simulink model "model"  (R2024b)
settings: Solver=ode4  StartTime=0.0  StopTime=tfinal  FixedStep=dt  RelTol=1e-3
values from neighbouring files (symbols this model uses):
  A_lateral = [YV , (W0+YP) , -U0+YR, g*cos(theta0), 0;         LV_DASH , LP_DASH , LR_DASH , 0 , 0;         NV_DASH , NP_DASH , NR_DASH , 0 , 0;         0 , 1 , tan(theta0) , 0 , 0;         0 , 0 , 1/cos(theta0) ,0 ,0]    [pre_simulink.m]
  A_longitudinal = [XU,XW,-W0,-g*cos(theta0);         ZU/(1-ZWD),ZW/(1-ZWD),(ZQ+U0)/(1-ZWD),-g*sin(theta0)/(1-ZWD);         MU+MWD*ZU/(1-ZWD),MW+MWD*ZW/(1-ZWD),MQ+MWD*(ZQ+U0)/(1-ZWD),-MWD*g*sin(theta0)/(1-ZWD);         0,0,1,0]    [pre_simulink.m]
  B_lateral = [YDA , YDR;          LDA_DASH , LDR_DASH;          NDA_DASH , NDR_DASH;          0 , 0;          0 , 0]    [pre_simulink.m]
  B_longitudinal = [XDE,XDTH ;         ZDE/(1-ZWD),ZDTH/(1-ZWD);         MDE+MWD*ZDE/(1-ZWD),MDTH+MWD*ZDTH/(1-ZWD);         0,0]    [pre_simulink.m]
  C_lateral = eye(5)    [pre_simulink.m]
  C_longitudinal = eye(4)    [pre_simulink.m]
  Controls_Matrix = [0,    XDE,   XDTH,      0 ... (first row only)    [aircraft_data_reader.m]
  D_lateral = zeros(5,2)    [pre_simulink.m]
  D_longitudinal = zeros(4,2)    [pre_simulink.m]
  dA = 0 *pi/180    (= 0)    [pre_simulink.m]
  dR = 0 *pi/180    (= 0)    [pre_simulink.m]
  dTH = 0    [pre_simulink.m]
  g = aircraft_data(52)    [aircraft_data_reader.m]
  Ixx = aircraft_data(53)    [aircraft_data_reader.m]
  Iyy = aircraft_data(54)    [aircraft_data_reader.m]
  Izz = aircraft_data(55)    [aircraft_data_reader.m]
  K = 1.5849    [pre_simulink.m]
  K_d_theta = 0.9182    [pre_simulink.m]
  K_i = 0.0332    [pre_simulink.m]
  m = aircraft_data(51)    [aircraft_data_reader.m]
  mg0 = m*g * [ sin(s0(8)) ; -cos(s0(8))*sin(s0(7)) ; -cos(s0(8))*cos(s0(7)) ]    [aircraft_data_reader.m]
  s0 = aircraft_data(4:15)    [aircraft_data_reader.m]
  States_Matrix = [XU,   0,   XW,    0,   0,   0,    0 ... (first row only)    [aircraft_data_reader.m]
  U0 = s0(1)    [aircraft_data_reader.m]
undefined symbols (not defined in the file or in its folder): A_lateral_1DOF, A_lateral_2DOF, A_lateral_3DOF_DR, A_lateral_3DOF_SP, A_longitudinal_lp, A_longitudinal_sp, alpha, B_lateral_1DOF, B_lateral_2DOF, B_lateral_3DOF_DR, B_lateral_3DOF_SP, B_longitudinal_lp, B_longitudinal_sp, beta, C_lateral_1DOF, C_lateral_2DOF, C_lateral_3DOF_DR, C_lateral_3DOF_SP, C_longitudinal_lp, C_longitudinal_sp, d_a, d_e, D_lateral_1DOF, D_lateral_2DOF, D_lateral_3DOF_DR, D_lateral_3DOF_SP, D_longitudinal_lp, D_longitudinal_sp, d_r, d_th, initial_states_bus, p, phi, psi, q, r, theta, v, VT, w, wdot, x, y, z
libraries: cstblocks x4, dspsigops x3, simulink_extras x1, shared6dof x1, aerolibasang x1
settings Model: Creator=ahmed  LastModifiedBy=ahmed
settings DebuggingCC: SignalInfNanChecking=warning  CheckMatrixSingularityMsg=warning  SignalLabelMismatchMsg=warning  StateNameClashWarn=warning

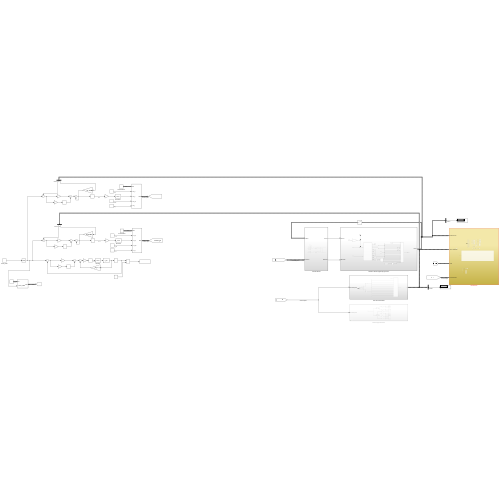
[thumbnail: Simulink's stored preview of the top-level diagram]
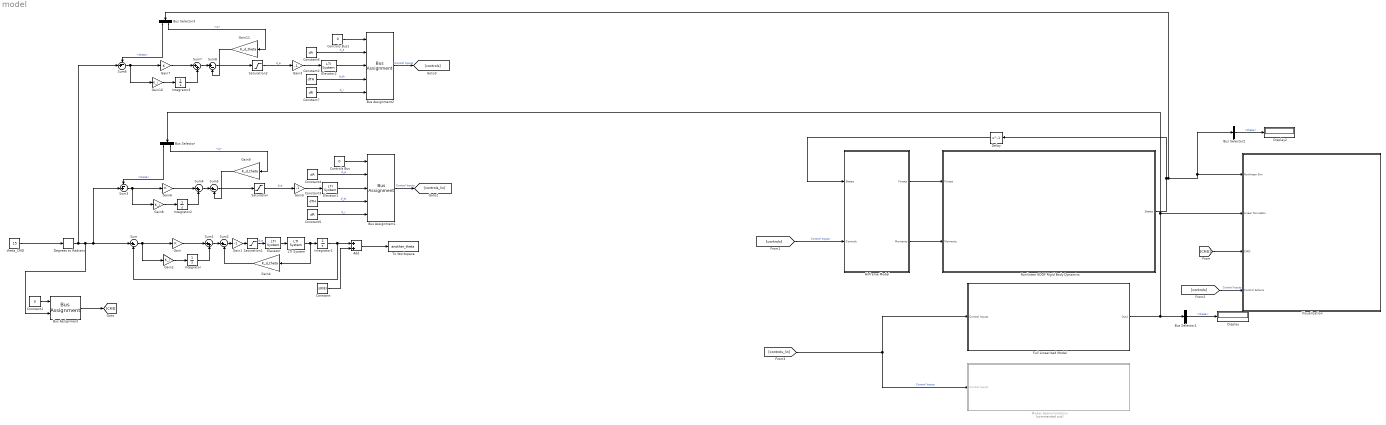
== system model ==
  Add : Sum
  Airframe Model : Subsystem
  Bus Assignment : BusAssignment  AssignedSignals=theta_CMD
  Bus Assignment1 : BusAssignment  AssignedSignals=d_a,d_e,d_th,d_r
  Bus Assignment2 : BusAssignment  AssignedSignals=d_a,d_e,d_th,d_r
  Bus Selector : BusSelector  OutputSignals=theta,q
  Bus Selector1 : BusSelector  OutputSignals=theta
  Bus Selector2 : BusSelector  OutputSignals=theta
  Bus Selector3 : BusSelector  OutputSignals=theta,q
  Constant : Constant  Value=s0(8)
  Constant1 : Constant  Value=0  OutDataTypeStr=Bus: CMD_States_bus_T
  Constant2 : Constant  Value=dTH
  Constant3 : Constant  Value=dTH
  Constant4 : Constant  Value=dA
  Constant5 : Constant  Value=dR
  Constant6 : Constant  Value=dA
  Constant7 : Constant  Value=dR
  Controls Bus : Constant  Value=0  OutDataTypeStr=Bus: Controls_bus_T
  Controls Bus1 : Constant  Value=0  OutDataTypeStr=Bus: Controls_bus_T
  Degrees to Radians : simulink_extras/Transformations/Degrees to Radians
  Delay : Delay  DelayLength=1  InitialCondition=initial_states_bus
  Display : Display
  Display2 : Display
  Elevator : cstblocks/LTI System  sys=servo  IC=[]  PadeOrder=0
  Elevator1 : cstblocks/LTI System  sys=servo  IC=[]  PadeOrder=0
  Elevator2 : cstblocks/LTI System  sys=servo  IC=[]  PadeOrder=0
  Full Linearized Model : Subsystem
  Gain : Gain  Gain=K
  Gain1 : Gain  Gain=-1
  Gain10 : Gain  Gain=K_i
  Gain11 : Gain  Gain=K_d_theta
  Gain2 : Gain  Gain=K_i
  Gain3 : Gain  Gain=-1
  Gain4 : Gain  Gain=K_d_theta
  Gain5 : Gain  Gain=-1
  Gain6 : Gain  Gain=K
  Gain7 : Gain  Gain=K
  Gain8 : Gain  Gain=K_i
  Gain9 : Gain  Gain=K_d_theta
  Integrator{,1..3} (4 alike) : Integrator
  LTI System : cstblocks/LTI System  sys=q_de  IC=[]  PadeOrder=0
  Modes Approximations : Subsystem  Commented=on
  Nonlinear 6DOF Rigid Body Dynamics : Subsystem
  Saturation : Saturate  UpperLimit=30*pi/180  LowerLimit=-30*pi/180
  Saturation1 : Saturate  UpperLimit=30*pi/180  LowerLimit=-30*pi/180
  Saturation2 : Saturate  UpperLimit=30*pi/180  LowerLimit=-30*pi/180
  Sum{,2,5,8} (4 alike) : Sum  Inputs=|+-
  Sum1 : Sum  Inputs=|++
  Sum3 : Sum  Inputs=-+|
  Sum4 : Sum  Inputs=|++
  Sum6 : Sum  Inputs=-+|
  Sum7 : Sum  Inputs=|++
  To Workspace : ToWorkspace  VariableName=another_theta  SaveFormat=Timeseries  SampleTime=-1
  Visualization : Subsystem
  theta_CMD : Constant  Value=15
  wires:
  Airframe Model/1(Forces) -> Nonlinear 6DOF Rigid Body Dynamics/1(Forces)
  Airframe Model/2(Moments) -> Nonlinear 6DOF Rigid Body Dynamics/2(Moments)
  Delay/1 -> Airframe Model/1(States)
  Bus Selector/1 -> Sum3/1  "<theta>"
  Gain1/1 -> Saturation1/1
  Integrator/1 -> Sum1/2
  Sum1/1 -> Sum2/1
  Gain2/1 -> Integrator/1
  Full Linearized Model/1(Out1) -> Visualization/2(Linear Simulator), Bus Selector/1, Bus Selector1/1
  Gain/1 -> Sum1/1
  LTI System/1 -> Gain4/1, Integrator1/1
  Integrator1/1 -> Sum/2, Add/1
  theta_CMD/1 -> Degrees to Radians/1
  Gain4/1 -> Sum2/2
  [controls] -> Airframe Model/2(Controls)  "Control Inputs"
  Constant4/1 -> Bus Assignment1/2  "d_a"
  Constant3/1 -> Bus Assignment1/4  "d_th"
  Elevator/1 -> LTI System/1
  Constant5/1 -> Bus Assignment1/5  "d_r"
  Controls Bus/1 -> Bus Assignment1/1
  Saturation/1 -> Gain5/1  "d_e"
  Gain5/1 -> Elevator1/1
  Elevator1/1 -> Bus Assignment1/3
  Bus Selector1/1 -> Display/1  "<theta>"
  Bus Selector2/1 -> Display2/1  "<theta>"
  [CMD] -> Visualization/3(CMD)
  Constant1/1 -> Bus Assignment/1
  Bus Assignment/1 -> [CMD]
  Constant/1 -> Add/2
  Add/1 -> To Workspace/1
  Bus Assignment1/1 -> [controls_lin]  "Control Inputs"
  [controls] -> Visualization/4(Control Actions)  "Control Inputs"
  Sum/1 -> Gain2/1, Gain/1
  Sum2/1 -> Gain1/1
  Gain8/1 -> Integrator2/1
  Sum5/1 -> Saturation/1
  Integrator2/1 -> Sum4/2
  Gain9/1 -> Sum5/2
  Gain6/1 -> Sum4/1
  Sum3/1 -> Gain8/1, Gain6/1
  Sum4/1 -> Sum5/1
  Saturation1/1 -> Elevator/1  "d_e"
  Bus Selector/2 -> Gain9/1  "<q>"
  Constant2/1 -> Bus Assignment2/4  "d_th"
  Gain7/1 -> Sum7/1
  Bus Assignment2/1 -> [controls]  "Control Inputs"
  Constant7/1 -> Bus Assignment2/5  "d_r"
  Integrator3/1 -> Sum7/2
  Bus Selector3/1 -> Sum6/1  "<theta>"
  Bus Selector3/2 -> Gain11/1  "<q>"
  Sum6/1 -> Gain10/1, Gain7/1
  Degrees to Radians/1 -> Sum6/2, Bus Assignment/2, Sum3/2, Sum/1
  Gain10/1 -> Integrator3/1
  Gain11/1 -> Sum8/2
  Elevator2/1 -> Bus Assignment2/3
  Sum7/1 -> Sum8/1
  Saturation2/1 -> Gain3/1  "d_e"
  Gain3/1 -> Elevator2/1
  Constant6/1 -> Bus Assignment2/2  "d_a"
  Nonlinear 6DOF Rigid Body Dynamics/1(States) -> Delay/1, Bus Selector2/1, Visualization/1(Nonlinear Sim), Bus Selector3/1
  Controls Bus1/1 -> Bus Assignment2/1
  Sum8/1 -> Saturation2/1
  [controls_lin] -> Full Linearized Model/1(Control Inputs), Modes Approximations/1(Control Inputs)  "Control Inputs"

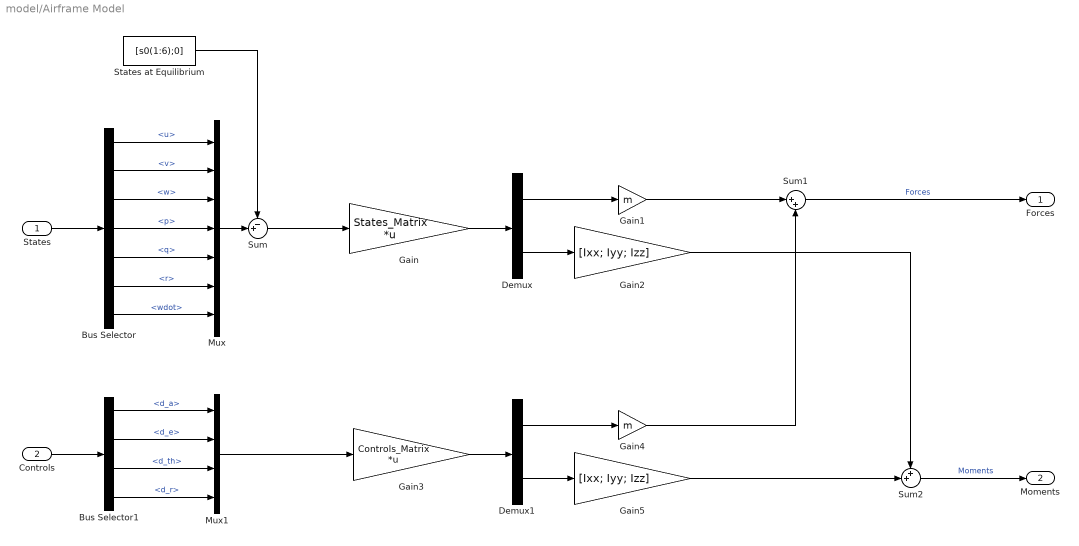
== system model/Airframe Model ==
  States : Inport  OutDataTypeStr=Bus: States_bus_T
  Controls : Inport  Port=2  OutDataTypeStr=Bus: Controls_bus_T
  Bus Selector : BusSelector  OutputSignals=u,v,w,p,q,r,wdot
  Bus Selector1 : BusSelector  OutputSignals=d_a,d_e,d_th,d_r
  Demux : Demux  Outputs=2
  Demux1 : Demux  Outputs=2
  Gain : Gain  Gain=States_Matrix  Multiplication=Matrix(K*u)
  Gain1 : Gain  Gain=m
  Gain2 : Gain  Gain=[Ixx; Iyy; Izz]
  Gain3 : Gain  Gain=Controls_Matrix  Multiplication=Matrix(K*u)
  Gain4 : Gain  Gain=m
  Gain5 : Gain  Gain=[Ixx; Iyy; Izz]
  Mux : Mux  Inputs=7
  Mux1 : Mux
  States at Equilibrium : Constant  Value=[s0(1:6);0]
  Sum : Sum  Inputs=-+|
  Sum1 : Sum  Inputs=|++
  Sum2 : Sum  Inputs=++|
  Forces : Outport
  Moments : Outport  Port=2
  wires:
  Sum1/1 -> Forces/1  "Forces"
  Sum2/1 -> Moments/1  "Moments"
  States/1 -> Bus Selector/1
  Bus Selector/2 -> Mux/2  "<v>"
  Bus Selector/1 -> Mux/1  "<u>"
  Bus Selector/3 -> Mux/3  "<w>"
  Bus Selector/4 -> Mux/4  "<p>"
  Bus Selector/5 -> Mux/5  "<q>"
  Bus Selector/6 -> Mux/6  "<r>"
  Bus Selector/7 -> Mux/7  "<wdot>"
  Mux/1 -> Sum/2
  States at Equilibrium/1 -> Sum/1
  Sum/1 -> Gain/1
  Gain/1 -> Demux/1
  Demux/1 -> Gain1/1
  Demux/2 -> Gain2/1
  Gain1/1 -> Sum1/1
  Gain2/1 -> Sum2/1
  Demux1/2 -> Gain5/1
  Gain3/1 -> Demux1/1
  Controls/1 -> Bus Selector1/1
  Bus Selector1/3 -> Mux1/3  "<d_th>"
  Bus Selector1/2 -> Mux1/2  "<d_e>"
  Bus Selector1/1 -> Mux1/1  "<d_a>"
  Bus Selector1/4 -> Mux1/4  "<d_r>"
  Mux1/1 -> Gain3/1
  Gain5/1 -> Sum2/2
  Demux1/1 -> Gain4/1
  Gain4/1 -> Sum1/2

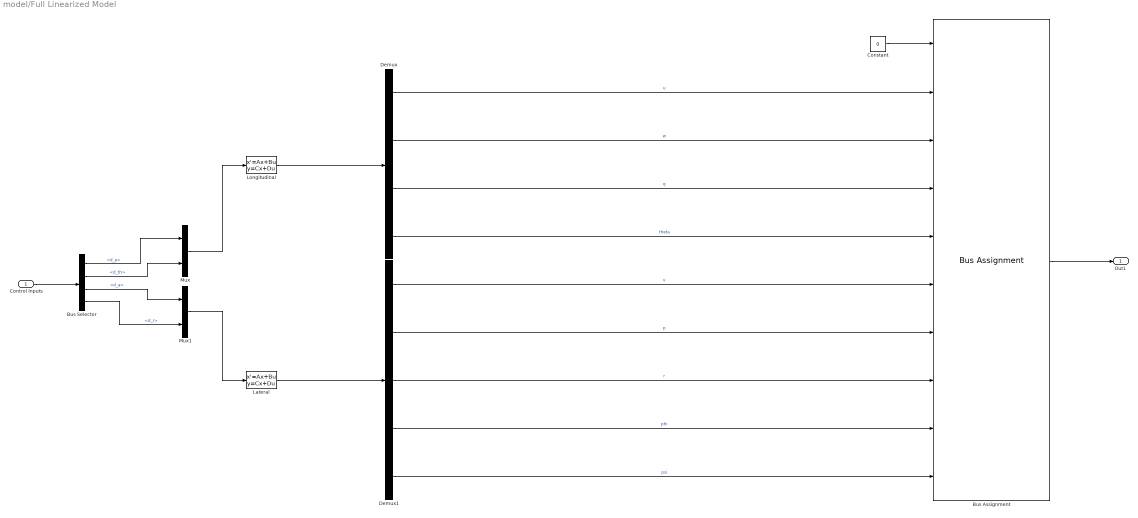
== system model/Full Linearized Model ==
  Control Inputs : Inport
  Bus Assignment : BusAssignment  AssignedSignals=u,w,q,theta,v,p,r,phi,psi
  Bus Selector : BusSelector  OutputSignals=d_e,d_th,d_a,d_r
  Constant : Constant  Value=0  OutDataTypeStr=Bus: Lin_States_bus_T
  Demux : Demux
  Demux1 : Demux  Outputs=5
  Lateral : StateSpace  A=A_lateral  B=B_lateral  C=C_lateral  D=D_lateral  InitialCondition=[s0(2); s0(4); s0(6); s0(7); s0(9)]
  Longitudinal : StateSpace  A=A_longitudinal  B=B_longitudinal  C=C_longitudinal  D=D_longitudinal  InitialCondition=[s0(1); s0(3); s0(5); s0(8)]
  Mux : Mux  Inputs=2
  Mux1 : Mux  Inputs=2
  Out1 : Outport
  wires:
  Bus Selector/4 -> Mux1/2  "<d_r>"
  Bus Selector/1 -> Mux/1  "<d_e>"
  Bus Selector/2 -> Mux/2  "<d_th>"
  Mux/1 -> Longitudinal/1
  Bus Selector/3 -> Mux1/1  "<d_a>"
  Longitudinal/1 -> Demux/1
  Control Inputs/1 -> Bus Selector/1
  Demux1/2 -> Bus Assignment/7  "p"
  Demux1/1 -> Bus Assignment/6  "v"
  Demux/4 -> Bus Assignment/5  "theta"
  Demux/2 -> Bus Assignment/3  "w"
  Demux/3 -> Bus Assignment/4  "q"
  Demux1/3 -> Bus Assignment/8  "r"
  Demux/1 -> Bus Assignment/2  "u"
  Demux1/4 -> Bus Assignment/9  "phi"
  Bus Assignment/1 -> Out1/1
  Lateral/1 -> Demux1/1
  Mux1/1 -> Lateral/1
  Constant/1 -> Bus Assignment/1
  Demux1/5 -> Bus Assignment/10  "psi"

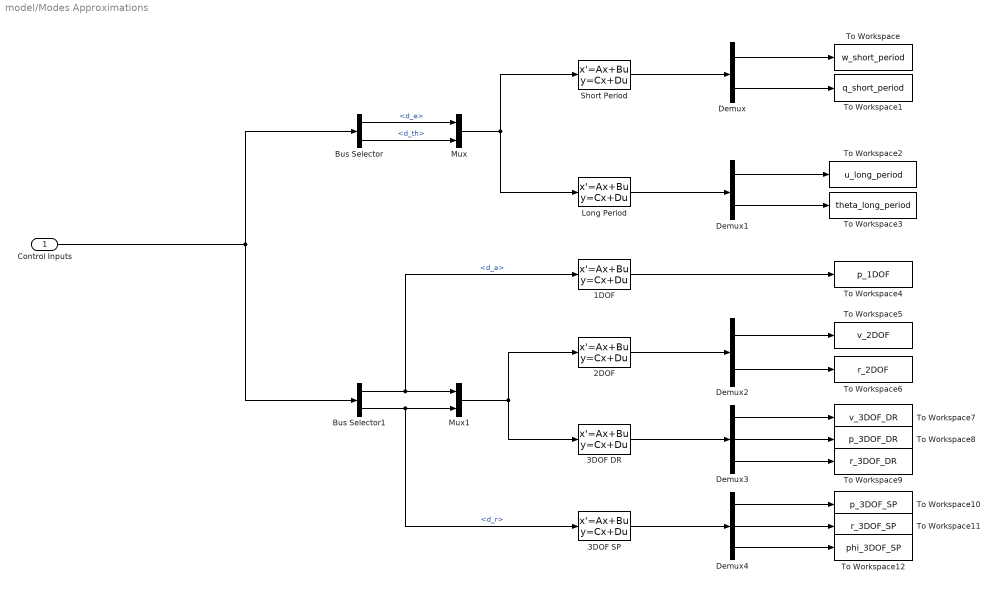
== system model/Modes Approximations ==
  Control Inputs : Inport
  1DOF : StateSpace  A=A_lateral_1DOF  B=B_lateral_1DOF  C=C_lateral_1DOF  D=D_lateral_1DOF  InitialCondition=s0(4)
  2DOF : StateSpace  A=A_lateral_2DOF  B=B_lateral_2DOF  C=C_lateral_2DOF  D=D_lateral_2DOF  InitialCondition=[s0(2); s0(6)]
  3DOF DR : StateSpace  A=A_lateral_3DOF_DR  B=B_lateral_3DOF_DR  C=C_lateral_3DOF_DR  D=D_lateral_3DOF_DR  InitialCondition=[s0(2); s0(4); s0(6)]
  3DOF SP : StateSpace  A=A_lateral_3DOF_SP  B=B_lateral_3DOF_SP  C=C_lateral_3DOF_SP  D=D_lateral_3DOF_SP  InitialCondition=[s0(4); s0(6); s0(7)]
  Bus Selector : BusSelector  OutputSignals=d_e,d_th
  Bus Selector1 : BusSelector  OutputSignals=d_a,d_r
  Demux : Demux  Outputs=2
  Demux1 : Demux  Outputs=2
  Demux2 : Demux  Outputs=2
  Demux3 : Demux  Outputs=3
  Demux4 : Demux  Outputs=3
  Long Period : StateSpace  A=A_longitudinal_lp  B=B_longitudinal_lp  C=C_longitudinal_lp  D=D_longitudinal_lp  InitialCondition=[s0(1); s0(8)]
  Mux : Mux  Inputs=2
  Mux1 : Mux  Inputs=2
  Short Period : StateSpace  A=A_longitudinal_sp  B=B_longitudinal_sp  C=C_longitudinal_sp  D=D_longitudinal_sp  InitialCondition=[s0(3); s0(5)]
  To Workspace : ToWorkspace  VariableName=w_short_period  SaveFormat=Timeseries  SampleTime=-1
  To Workspace1 : ToWorkspace  VariableName=q_short_period  SaveFormat=Timeseries  SampleTime=-1
  To Workspace10 : ToWorkspace  VariableName=p_3DOF_SP  SaveFormat=Timeseries  SampleTime=-1
  To Workspace11 : ToWorkspace  VariableName=r_3DOF_SP  SaveFormat=Timeseries  SampleTime=-1
  To Workspace12 : ToWorkspace  VariableName=phi_3DOF_SP  SaveFormat=Timeseries  SampleTime=-1
  To Workspace2 : ToWorkspace  VariableName=u_long_period  SaveFormat=Timeseries  SampleTime=-1
  To Workspace3 : ToWorkspace  VariableName=theta_long_period  SaveFormat=Timeseries  SampleTime=-1
  To Workspace4 : ToWorkspace  VariableName=p_1DOF  SaveFormat=Timeseries  SampleTime=-1
  To Workspace5 : ToWorkspace  VariableName=v_2DOF  SaveFormat=Timeseries  SampleTime=-1
  To Workspace6 : ToWorkspace  VariableName=r_2DOF  SaveFormat=Timeseries  SampleTime=-1
  To Workspace7 : ToWorkspace  VariableName=v_3DOF_DR  SaveFormat=Timeseries  SampleTime=-1
  To Workspace8 : ToWorkspace  VariableName=p_3DOF_DR  SaveFormat=Timeseries  SampleTime=-1
  To Workspace9 : ToWorkspace  VariableName=r_3DOF_DR  SaveFormat=Timeseries  SampleTime=-1
  wires:
  Demux4/2 -> To Workspace11/1
  Bus Selector1/1 -> 1DOF/1, Mux1/1  "<d_a>"
  Demux1/1 -> To Workspace2/1
  Demux3/2 -> To Workspace8/1
  Demux3/3 -> To Workspace9/1
  Demux2/1 -> To Workspace5/1
  Demux2/2 -> To Workspace6/1
  3DOF SP/1 -> Demux4/1
  Mux1/1 -> 3DOF DR/1, 2DOF/1
  Short Period/1 -> Demux/1
  Demux3/1 -> To Workspace7/1
  Demux4/1 -> To Workspace10/1
  Demux1/2 -> To Workspace3/1
  Control Inputs/1 -> Bus Selector/1, Bus Selector1/1
  Long Period/1 -> Demux1/1
  Demux4/3 -> To Workspace12/1
  1DOF/1 -> To Workspace4/1
  Bus Selector1/2 -> 3DOF SP/1, Mux1/2  "<d_r>"
  3DOF DR/1 -> Demux3/1
  Demux/1 -> To Workspace/1
  2DOF/1 -> Demux2/1
  Bus Selector/2 -> Mux/2  "<d_th>"
  Mux/1 -> Long Period/1, Short Period/1
  Demux/2 -> To Workspace1/1
  Bus Selector/1 -> Mux/1  "<d_e>"

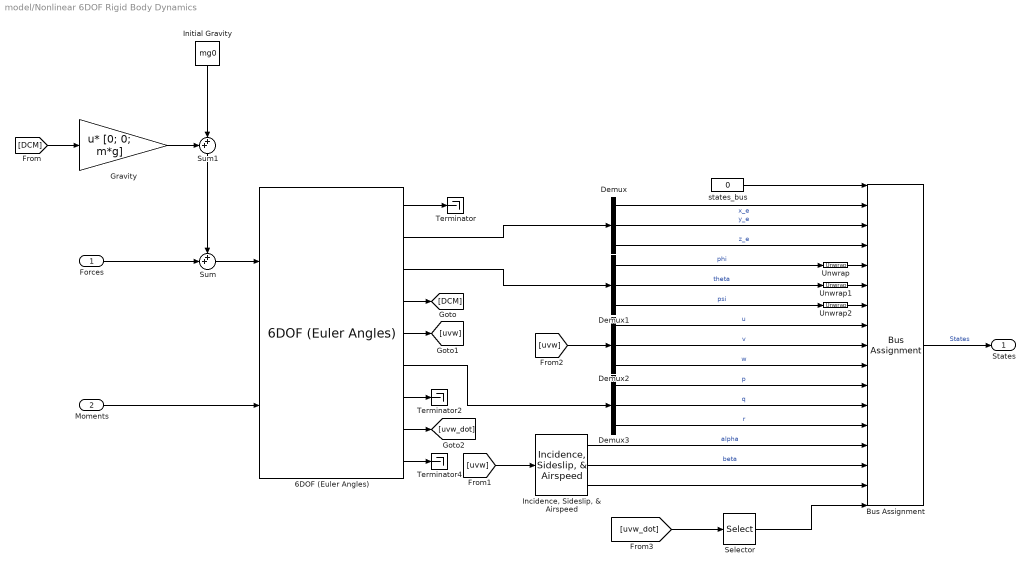
== system model/Nonlinear 6DOF Rigid Body Dynamics ==
  Forces : Inport
  Moments : Inport  Port=2
  6DOF (Euler Angles) : shared6dof/6DOF (Euler Angles)  units=English (Velocity in ft/s)  mtype=Fixed  rep=Euler Angles  xme_0=s0(10:12)  Vm_0=s0(1:3)  eul_0=s0(7:9)  pm_0=s0(4:6)  mass_0=m  mass_e=0.5  mass_f=2.0  inertia=I  inertia_e=eye(3)  inertia_f=2*eye(3)  k_quat=1.0  vre_flag=on  abi_flag=on  aMode=0  xme_statename=''  Vm_statename=''  eul_statename=''  quat_statename=''  pm_statename=''  mass_statename=''
  Bus Assignment : BusAssignment  AssignedSignals=x,y,z,phi,theta,psi,u,v,w,p,q,r,alpha,beta,VT,wdot
  Demux{,1..3} (4 alike) : Demux  Outputs=3
  Gravity : Gain  Gain=[0; 0; m*g]  Multiplication=Matrix(u*K)
  "Incidence, Sideslip, & Airspeed" : aerolibasang/Incidence, Sideslip, & Airspeed
  Initial Gravity : Constant  Value=mg0
  Selector : Selector  InputPortWidth=3  IndexOptions=Index vector (dialog)  Indices=3  OutputSizes=1
  Sum : Sum  Inputs=++|
  Sum1 : Sum  Inputs=++|
  Terminator : Terminator
  Terminator2 : Terminator
  Terminator4 : Terminator
  Unwrap : dspsigops/Unwrap  tol=pi  running=off
  Unwrap1 : dspsigops/Unwrap  tol=pi  running=off
  Unwrap2 : dspsigops/Unwrap  tol=pi  running=off
  states_bus : Constant  Value=0  OutDataTypeStr=Bus: States_bus_T  SampleTime=-1
  States : Outport  OutDataTypeStr=Bus: States_bus_T
  wires:
  Bus Assignment/1 -> States/1  "States"
  Demux1/2 -> Unwrap1/1  "theta"
  Demux3/2 -> Bus Assignment/12  "q"
  6DOF (Euler Angles)/7 -> Terminator2/1
  6DOF (Euler Angles)/1 -> Terminator/1
  6DOF (Euler Angles)/3 -> Demux1/1
  states_bus/1 -> Bus Assignment/1
  Forces/1 -> Sum/2
  6DOF (Euler Angles)/6 -> Demux3/1
  6DOF (Euler Angles)/8 -> [uvw_dot]
  Demux2/2 -> Bus Assignment/9  "v"
  Demux1/3 -> Unwrap2/1  "psi"
  Demux3/3 -> Bus Assignment/13  "r"
  Demux2/1 -> Bus Assignment/8  "u"
  Demux2/3 -> Bus Assignment/10  "w"
  6DOF (Euler Angles)/2 -> Demux/1
  Demux/3 -> Bus Assignment/4  "z_e"
  Demux1/1 -> Unwrap/1  "phi"
  Demux/2 -> Bus Assignment/3  "y_e"
  Demux/1 -> Bus Assignment/2  "x_e"
  6DOF (Euler Angles)/9 -> Terminator4/1
  Demux3/1 -> Bus Assignment/11  "p"
  6DOF (Euler Angles)/4 -> [DCM]
  Unwrap/1 -> Bus Assignment/5
  Unwrap1/1 -> Bus Assignment/6
  Unwrap2/1 -> Bus Assignment/7
  [DCM] -> Gravity/1
  Gravity/1 -> Sum1/1
  Initial Gravity/1 -> Sum1/2
  Sum1/1 -> Sum/1
  Sum/1 -> 6DOF (Euler Angles)/1
  6DOF (Euler Angles)/5 -> [uvw]
  [uvw] -> "Incidence, Sideslip, & Airspeed"/1
  "Incidence, Sideslip, & Airspeed"/3 -> Bus Assignment/16
  "Incidence, Sideslip, & Airspeed"/2 -> Bus Assignment/15  "beta"
  "Incidence, Sideslip, & Airspeed"/1 -> Bus Assignment/14  "alpha"
  [uvw] -> Demux2/1
  Moments/1 -> 6DOF (Euler Angles)/2
  [uvw_dot] -> Selector/1
  Selector/1 -> Bus Assignment/17

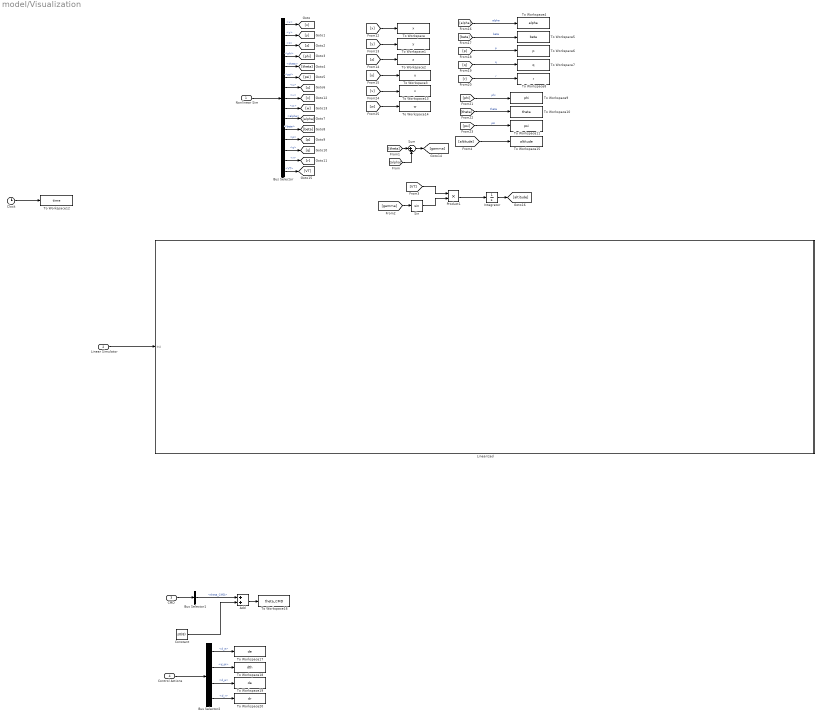
== system model/Visualization ==
  Nonlinear Sim : Inport
  Linear Simulator : Inport  Port=2
  CMD : Inport  Port=3
  Control Actions : Inport  Port=4
  Add : Sum
  Bus Selector : BusSelector  OutputSignals=x,y,z,phi,theta,psi,u,v,w,alpha,beta,p,q,r,VT
  Bus Selector1 : BusSelector  OutputSignals=theta_CMD
  Bus Selector2 : BusSelector  OutputSignals=d_e,d_th,d_a,d_r
  Clock : Clock
  Constant : Constant  Value=s0(8)
  Integrator : Integrator
  Linearized : Subsystem
  Product1 : Product
  Sin : Trigonometry
  Sum : Sum  Inputs=|+-
  To Workspace : ToWorkspace  VariableName=x  SaveFormat=Timeseries  SampleTime=-1
  To Workspace1 : ToWorkspace  VariableName=y  SaveFormat=Timeseries  SampleTime=-1
  To Workspace10 : ToWorkspace  VariableName=theta  SaveFormat=Timeseries  SampleTime=-1
  To Workspace11 : ToWorkspace  VariableName=psi  SaveFormat=Timeseries  SampleTime=-1
  To Workspace12 : ToWorkspace  VariableName=time  SaveFormat=Timeseries  SampleTime=-1
  To Workspace13 : ToWorkspace  VariableName=v  SaveFormat=Timeseries  SampleTime=-1
  To Workspace14 : ToWorkspace  VariableName=w  SaveFormat=Timeseries  SampleTime=-1
  To Workspace15 : ToWorkspace  VariableName=altitude  SaveFormat=Timeseries  SampleTime=-1
  To Workspace16 : ToWorkspace  VariableName=theta_CMD  SaveFormat=Timeseries  SampleTime=-1
  To Workspace17 : ToWorkspace  VariableName=de  SaveFormat=Timeseries  SampleTime=-1
  To Workspace18 : ToWorkspace  VariableName=dth  SaveFormat=Timeseries  SampleTime=-1
  To Workspace19 : ToWorkspace  VariableName=da  SaveFormat=Timeseries  SampleTime=-1
  To Workspace2 : ToWorkspace  VariableName=z  SaveFormat=Timeseries  SampleTime=-1
  To Workspace20 : ToWorkspace  VariableName=dr  SaveFormat=Timeseries  SampleTime=-1
  To Workspace3 : ToWorkspace  VariableName=u  SaveFormat=Timeseries  SampleTime=-1
  To Workspace4 : ToWorkspace  VariableName=alpha  SaveFormat=Timeseries  SampleTime=-1
  To Workspace5 : ToWorkspace  VariableName=beta  SaveFormat=Timeseries  SampleTime=-1
  To Workspace6 : ToWorkspace  VariableName=p  SaveFormat=Timeseries  SampleTime=-1
  To Workspace7 : ToWorkspace  VariableName=q  SaveFormat=Timeseries  SampleTime=-1
  To Workspace8 : ToWorkspace  VariableName=r  SaveFormat=Timeseries  SampleTime=-1
  To Workspace9 : ToWorkspace  VariableName=phi  SaveFormat=Timeseries  SampleTime=-1
  wires:
  Bus Selector/6 -> [psi]  "<psi>"
  Bus Selector/1 -> [x]  "<x>"
  Bus Selector/7 -> [u]  "<u>"
  Bus Selector/4 -> [phi]  "<phi>"
  Bus Selector/10 -> [alpha]  "<alpha>"
  Bus Selector/14 -> [r]  "<r>"
  Bus Selector/11 -> [beta]  "<beta>"
  Bus Selector/5 -> [theta]  "<theta>"
  Bus Selector/13 -> [q]  "<q>"
  Bus Selector/12 -> [p]  "<p>"
  Bus Selector/2 -> [y]  "<y>"
  Bus Selector/3 -> [z]  "<z>"
  Nonlinear Sim/1 -> Bus Selector/1
  [x] -> To Workspace/1
  [y] -> To Workspace1/1
  [z] -> To Workspace2/1
  [u] -> To Workspace3/1
  Clock/1 -> To Workspace12/1
  [phi] -> To Workspace9/1  "phi"
  [theta] -> To Workspace10/1  "theta"
  [psi] -> To Workspace11/1  "psi"
  [alpha] -> To Workspace4/1  "alpha"
  [beta] -> To Workspace5/1  "beta"
  [p] -> To Workspace6/1  "p"
  [q] -> To Workspace7/1  "q"
  [r] -> To Workspace8/1  "r"
  [v] -> To Workspace13/1
  Bus Selector/8 -> [v]  "<v>"
  Bus Selector/9 -> [w]  "<w>"
  [w] -> To Workspace14/1
  [theta] -> Sum/1
  [alpha] -> Sum/2
  Sum/1 -> [gamma]
  [gamma] -> Sin/1
  Bus Selector/15 -> [VT]  "<VT>"
  [VT] -> Product1/1
  Sin/1 -> Product1/2
  Product1/1 -> Integrator/1
  Integrator/1 -> [altitude]
  [altitude] -> To Workspace15/1
  Linear Simulator/1 -> Linearized/1(In4)
  CMD/1 -> Bus Selector1/1
  Bus Selector1/1 -> Add/1  "<theta_CMD>"
  Constant/1 -> Add/2
  Add/1 -> To Workspace16/1
  Control Actions/1 -> Bus Selector2/1
  Bus Selector2/1 -> To Workspace17/1  "<d_e>"
  Bus Selector2/2 -> To Workspace18/1  "<d_th>"
  Bus Selector2/3 -> To Workspace19/1  "<d_a>"
  Bus Selector2/4 -> To Workspace20/1  "<d_r>"

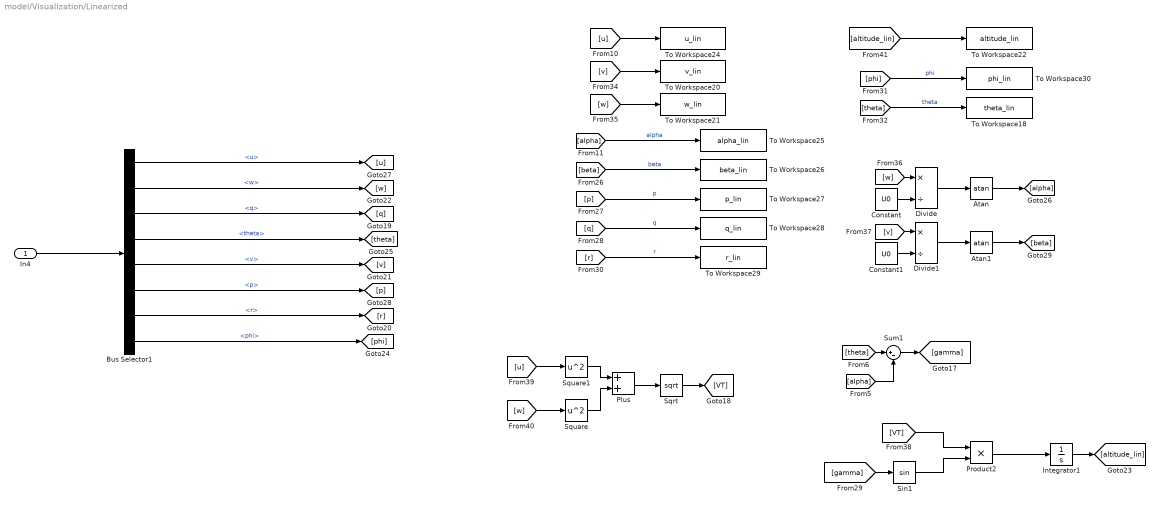
== system model/Visualization/Linearized ==
  In4 : Inport
  Atan : Trigonometry  Operator=atan
  Atan1 : Trigonometry  Operator=atan
  Bus Selector1 : BusSelector  OutputSignals=u,w,q,theta,v,p,r,phi
  Constant : Constant  Value=U0
  Constant1 : Constant  Value=U0
  Divide : Product  Inputs=*/
  Divide1 : Product  Inputs=*/
  Integrator1 : Integrator
  Plus : Sum
  Product2 : Product
  Sin1 : Trigonometry
  Sqrt : Sqrt
  Square : Math  Operator=square
  Square1 : Math  Operator=square
  Sum1 : Sum  Inputs=|+-
  To Workspace18 : ToWorkspace  VariableName=theta_lin  SaveFormat=Timeseries  SampleTime=-1
  To Workspace20 : ToWorkspace  VariableName=v_lin  SaveFormat=Timeseries  SampleTime=-1
  To Workspace21 : ToWorkspace  VariableName=w_lin  SaveFormat=Timeseries  SampleTime=-1
  To Workspace22 : ToWorkspace  VariableName=altitude_lin  SaveFormat=Timeseries  SampleTime=-1
  To Workspace24 : ToWorkspace  VariableName=u_lin  SaveFormat=Timeseries  SampleTime=-1
  To Workspace25 : ToWorkspace  VariableName=alpha_lin  SaveFormat=Timeseries  SampleTime=-1
  To Workspace26 : ToWorkspace  VariableName=beta_lin  SaveFormat=Timeseries  SampleTime=-1
  To Workspace27 : ToWorkspace  VariableName=p_lin  SaveFormat=Timeseries  SampleTime=-1
  To Workspace28 : ToWorkspace  VariableName=q_lin  SaveFormat=Timeseries  SampleTime=-1
  To Workspace29 : ToWorkspace  VariableName=r_lin  SaveFormat=Timeseries  SampleTime=-1
  To Workspace30 : ToWorkspace  VariableName=phi_lin  SaveFormat=Timeseries  SampleTime=-1
  wires:
  [u] -> Square1/1
  [alpha] -> To Workspace25/1  "alpha"
  [r] -> To Workspace29/1  "r"
  [alpha] -> Sum1/2
  Sqrt/1 -> [VT]
  Constant/1 -> Divide/2
  [w] -> Divide/1
  Atan/1 -> [alpha]
  Product2/1 -> Integrator1/1
  Sin1/1 -> Product2/2
  [p] -> To Workspace27/1  "p"
  [w] -> To Workspace21/1
  Integrator1/1 -> [altitude_lin]
  [beta] -> To Workspace26/1  "beta"
  Atan1/1 -> [beta]
  [v] -> Divide1/1
  [q] -> To Workspace28/1  "q"
  Plus/1 -> Sqrt/1
  [theta] -> To Workspace18/1  "theta"
  [altitude_lin] -> To Workspace22/1
  Divide/1 -> Atan/1
  In4/1 -> Bus Selector1/1
  [gamma] -> Sin1/1
  [VT] -> Product2/1
  Square/1 -> Plus/2
  Constant1/1 -> Divide1/2
  Square1/1 -> Plus/1
  [v] -> To Workspace20/1
  Divide1/1 -> Atan1/1
  [w] -> Square/1
  [phi] -> To Workspace30/1  "phi"
  [u] -> To Workspace24/1
  Sum1/1 -> [gamma]
  [theta] -> Sum1/1
  Bus Selector1/8 -> [phi]  "<phi>"
  Bus Selector1/4 -> [theta]  "<theta>"
  Bus Selector1/7 -> [r]  "<r>"
  Bus Selector1/3 -> [q]  "<q>"
  Bus Selector1/6 -> [p]  "<p>"
  Bus Selector1/2 -> [w]  "<w>"
  Bus Selector1/5 -> [v]  "<v>"
  Bus Selector1/1 -> [u]  "<u>"
